simulink model "DCMotor_Final"  (R2021b)
settings: Solver=VariableStepAuto  StartTime=0.0  StopTime=10.0  RelTol=1e-3
InitFcn:
  | dcMotorParams
values from neighbouring files (symbols this model uses):
  b = 0.1    [dcMotorParams.m]
  J = 0.01    [dcMotorParams.m]
  K_EMF = 0.01    [dcMotorParams.m]
  K_T = 0.01    [dcMotorParams.m]
  L = 0.5    [dcMotorParams.m]
  R = 1    [dcMotorParams.m]
settings Model: Creator=ecosg  LastModifiedBy=ecosg

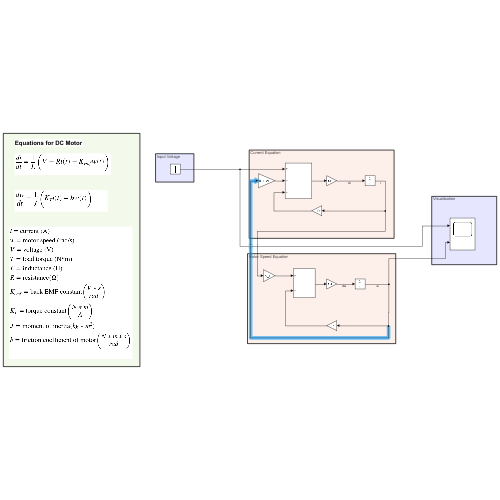
[thumbnail: Simulink's stored preview of the top-level diagram]
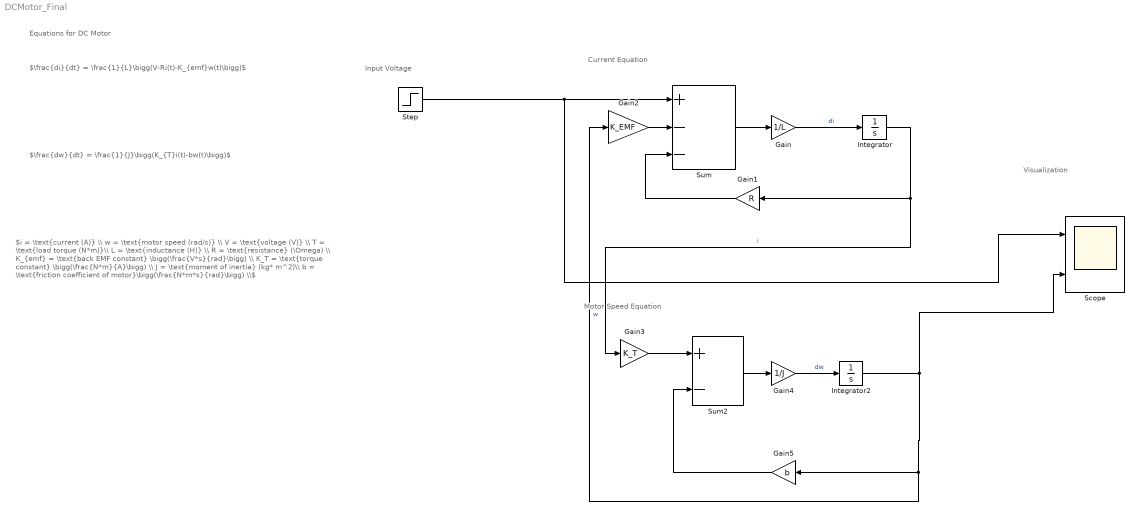
== system DCMotor_Final ==
  note: Visualization
  note: $i = \text{current (A)} \\ w = \text{motor speed (rad/s)} \\ V = \text{voltage (V)} \\ T = \text{load torque (N*m)}\\ L = \text{inductance (H)} \\ R = \text{resistance} (\Omega) \\ K_{emf} = \text{back EMF constant} \bigg(\frac{V*s}{rad}\bigg) \\ K_T = \text{torque constant} \bigg(\frac{N*m}{A}\bigg) \\ J = \text{moment of inertia} (kg* m^2)\\ b = \text{friction coefficient of motor}\bigg(\frac{N*m*s}{rad}\bigg) \\$
  note: $\frac{di}{dt} = \frac{1}{L}\bigg(V-Ri(t)-K_{emf}w(t)\bigg)$
  note: Equations for DC Motor
  note: Input Voltage
  note: $\frac{dw}{dt} = \frac{1}{J}\bigg(K_{T}i(t)-bw(t)\bigg)$
  note: Motor Speed Equation
  note: Current Equation
  Gain : Gain  Gain=1/L
  Gain1 : Gain  Gain=R
  Gain2 : Gain  Gain=K_EMF
  Gain3 : Gain  Gain=K_T
  Gain4 : Gain  Gain=1/J
  Gain5 : Gain  Gain=b
  Integrator : Integrator
  Integrator2 : Integrator
  Scope : Scope  NumInputPorts=2
  Step : Step  After=10  SampleTime=0
  Sum : Sum  Inputs=+--
  Sum2 : Sum  Inputs=+-
  wires:
  Step/1 -> Scope/1, Sum/1
  Gain/1 -> Integrator/1  "di"
  Sum/1 -> Gain/1
  Integrator/1 -> Gain3/1, Gain1/1  "i"
  Gain1/1 -> Sum/3
  Gain5/1 -> Sum2/2
  Gain4/1 -> Integrator2/1  "dw"
  Sum2/1 -> Gain4/1
  Integrator2/1 -> Scope/2, Gain2/1, Gain5/1  "w"
  Gain2/1 -> Sum/2
  Gain3/1 -> Sum2/1
